simulink model "newAutocar"  (R2021b)
settings: Solver=VariableStepAuto  StartTime=0.0  StopTime=15  RelTol=1e-3
values from neighbouring files (symbols this model uses):
  Cf = 19000    [new_ref1.mat]
  Cr = 33000    [new_ref1.mat]
  Iz = 3344    [new_ref1.mat]
  m = 2050    [new_ref1.mat]
  Vx = 15    [new_ref1.mat]
undefined symbols (not defined in the file or in its folder): lf, lr
libraries: mpclib x1
settings Model: Creator=The MathWorks, Inc.  LastModifiedBy=Advait
settings SolverCC: AlgebraicLoopSolver=TrustRegion
settings DataIOCC: ReturnWorkspaceOutputs=off
settings DebuggingCC: SFMachineParentedDataDiag=warning  ArithmeticOperatorsInVariantConditions=warning
settings SFSimCC: SimUseLocalCustomCode=off  CustomCodeUndefinedFunction=UseInterfaceOnly
settings RTWCC: RTWUseLocalCustomCode=off
settings CodeAppCC: StateflowObjectComments=on
settings SimscapeCC: SimscapeNormalizeSystem=off

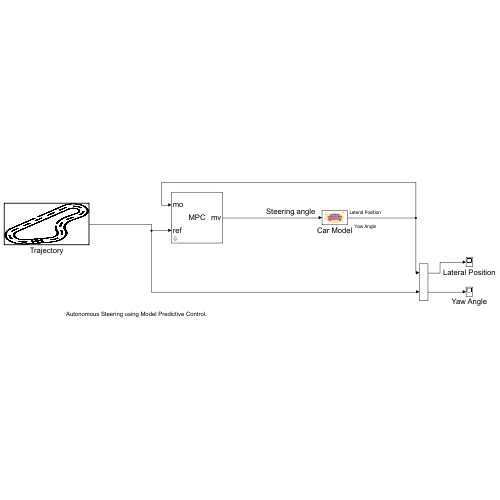
[thumbnail: Simulink's stored preview of the top-level diagram]
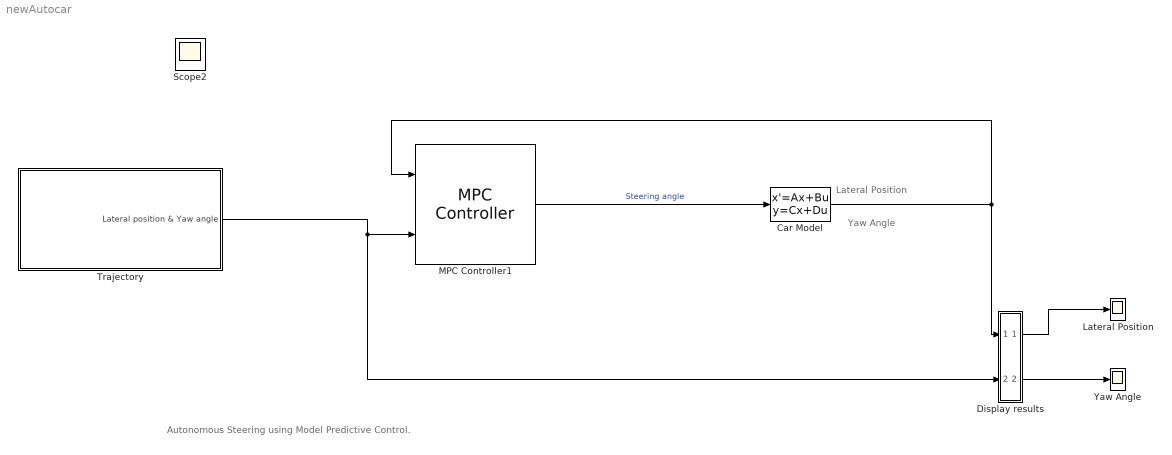
== system newAutocar ==
  note: Yaw Angle
  note: Lateral Position
  note: Autonomous Steering using Model Predictive Control.
  Car Model : StateSpace  A="[-(2*Cf+2*Cr)/(m*Vx), -Vx-(2*Cf*lf-2*Cr*lr)/m/Vx;  -(2*Cf*lf-2*Cr*lr)/Iz/Vx, -(2*Cf*lf^2+2*Cr*lr^2)/(Iz*Vx)]"  B=[2*Cf/m ; 2*Cf*lf/Iz]  C=[1,0;0,1]  D=[0;0]  InitialCondition=0
      mask Display: image('C:\Users\Advait\Downloads\icons8-car-50.png'); % Use "Edit Image" on toolstrip to change.
  Display results : Subsystem
  Lateral Position : Scope
  MPC Controller1 : mpclib/MPC Controller  SCDEnableBlockLinearizationSpecification=on  mpcobj=mpc1  is_multiple=0  enable_value=0  return_u0=off  updateMPCinCallerWorkspace=on  md_inport=off  mv_inport=off  uref_inport=off  return_cost=off  return_mvseq=off  return_qpstatus=off  return_xseq=off  return_state=off  return_ovseq=off  state_inport=off  umin_inport=off  umax_inport=off  ymin_inport=off  ymax_inport=off  cc_inport=off  ywt_inport=off  uwt_inport=off  duwt_inport=off  rhoeps_inport=off  pm_inport=off  MaximumP=10  HorizonChoice=FixedHorizon  n_ts=0.05  n_p=10  n_mv=1  n_md=0  n_ud=0  n_mo=2  n_uo=0  BlockDataType=double  SampleTimeInherited=off  switch_inport=off
  Trajectory : Subsystem  TreatAsAtomicUnit=on
      mask Display: image('C:\Users\Advait\Downloads\race-track.png'); % Use "Edit Image" on toolstrip to change.
  Yaw Angle : Scope
  Scope2 : Scope
  wires:
  MPC Controller1/1 -> Car Model/1  "Steering angle"
  Car Model/1 -> MPC Controller1/1, Display results/1(Outputs)
  Trajectory/1(Lateral position & Yaw angle) -> MPC Controller1/2, Display results/2(References)
  Display results/2(Out1) -> Yaw Angle/1
  Display results/1(Out2) -> Lateral Position/1

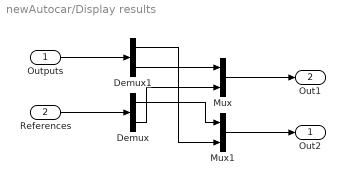
== system newAutocar/Display results ==
  Outputs : Inport
  References : Inport  Port=2
  Demux : Demux  Outputs=2
  Demux1 : Demux  Outputs=2
  Mux : Mux  Inputs=2
  Mux1 : Mux  Inputs=2
  Out2 : Outport  VectorParamsAs1DForOutWhenUnconnected=off
  Out1 : Outport  Port=2  VectorParamsAs1DForOutWhenUnconnected=off
  wires:
  Demux/2 -> Mux/2
  Mux/1 -> Out1/1
  Demux1/1 -> Mux1/2
  Demux/1 -> Mux1/1
  Demux1/2 -> Mux/1
  Mux1/1 -> Out2/1
  Outputs/1 -> Demux1/1
  References/1 -> Demux/1

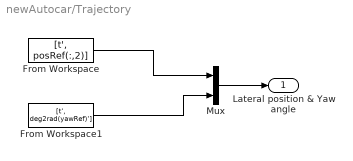
== system newAutocar/Trajectory ==
  From Workspace : FromWorkspace  VariableName=[t', posRef(:,2)]  SampleTime=0.1
  From Workspace1 : FromWorkspace  VariableName=[t', deg2rad(yawRef)']  SampleTime=0.1
  Mux : Mux  Inputs=2
  Lateral position & Yaw angle : Outport  VectorParamsAs1DForOutWhenUnconnected=off
  wires:
  From Workspace/1 -> Mux/1
  From Workspace1/1 -> Mux/2
  Mux/1 -> Lateral position & Yaw angle/1
